simulink model "Plant"  (R2022b)
settings: Solver=FixedStepAuto  StartTime=start_time  StopTime=end_time  FixedStep=PLANT_CONST.dt  RelTol=1e-3  EnableMultiTasking=on
values from neighbouring files (symbols this model uses):
  PLANT_EXPORT = Simulink.Parameter(PLANT_EXPORT_VALUE)    [plant_model_init.m]
undefined symbols (not defined in the file or in its folder): acc_x, acc_x_O, acc_y, acc_y_O, acc_z, acc_z_O, alt, alt_0, DiscIntNeverNeededParam, fixType, gyr_x, gyr_y, gyr_z, h_R, hAcc, height, lat, lon, M_BO, M_OB, mag_x, mag_y, mag_z, numSV, phi, PLANT_CONST, psi, quat, rot_x_B, rot_y_B, rot_z_B, sAcc, Sensor_Model, temprature, theta, timestamp, vAcc, vel_x_O, vel_y_O, vel_z_O, velD, velE, velN, x_R, y_R
libraries: FMT_Model_Lib x9, dspsrcs4 x5, simulink_extras x1, autolibshared x1, simulink x1
(part 1 of 2)
settings Model: Creator=19114  LastModifiedBy=19114
settings OptimizationCC: DefaultParameterBehavior=Inlined  EnhancedBackFolding=on  PassReuseOutputArgsAs=Individual arguments  ZeroExternalMemoryAtStartup=off  ZeroInternalMemoryAtStartup=off  OptimizeBlockOrder=speed  DifferentSizesBufferReuse=on  OptimizationCustomize=off  EfficientTunableParamExpr=on
settings DebuggingCC: ParameterTunabilityLossMsg=error
settings SFSimCC: MATLABDynamicMemAlloc=off
settings RTWCC: Description=Embedded Coder  SystemTargetFile=ert.tlc  TemplateMakefile=ert_default_tmf
settings CodeAppCC: ForceParamTrailComments=on  IgnoreCustomStorageClasses=off  OperatorAnnotations=on  SimulinkDataObjDesc=on  SFDataObjDesc=on  InsertBlockDesc=on
settings ERTTargetCC: TargetLangStandard=C99 (ISO)  GenerateSampleERTMain=on  InlinedParameterPlacement=NonHierarchical  ERTCustomFileTemplate=example_file_process.tlc

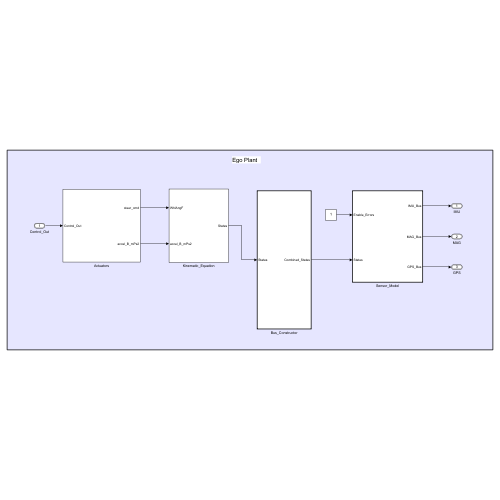
[thumbnail: Simulink's stored preview of the top-level diagram]
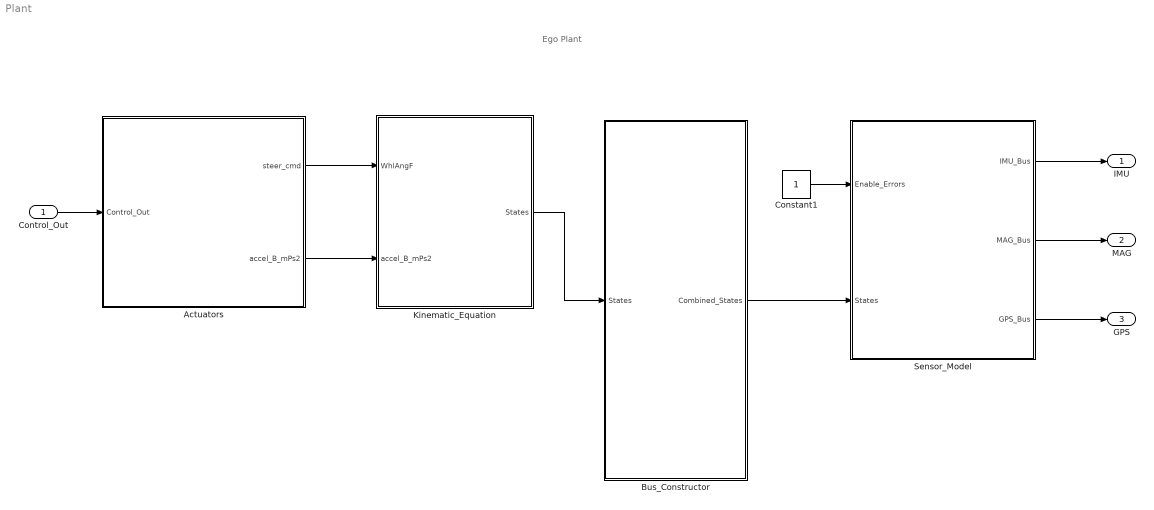
== system Plant ==
  note: Ego Plant
  Control_Out : Inport  OutDataTypeStr=Bus: Control_Out_Bus
  Actuators : Subsystem
  Bus_Constructor : Subsystem  TreatAsAtomicUnit=on  mask{lat_0=0.65673, lon_0=-2.1361, hgt_0=0}
      mask prompts: lat_0 "init latitude (rad)"; lon_0 "init lontitude (rad)"; hgt_0 "init height (m)"
  Constant1 : Constant  OutDataTypeStr=Inherit: Inherit via back propagation
  Kinematic_Equation : Subsystem
  Sensor_Model : Subsystem  TreatAsAtomicUnit=on
  IMU : Outport  OutDataTypeStr=Bus: IMU_Bus  VectorParamsAs1DForOutWhenUnconnected=off
  MAG : Outport  Port=2  OutDataTypeStr=Bus: MAG_Bus  VectorParamsAs1DForOutWhenUnconnected=off
  GPS : Outport  Port=3  OutDataTypeStr=Bus: GPS_uBlox_Bus  VectorParamsAs1DForOutWhenUnconnected=off
  wires:
  Control_Out/1 -> Actuators/1(Control_Out)
  Actuators/1(steer_cmd) -> Kinematic_Equation/1(WhlAngF)
  Kinematic_Equation/1(States) -> Bus_Constructor/1(States)
  Actuators/2(accel_B_mPs2) -> Kinematic_Equation/2(accel_B_mPs2)
  Constant1/1 -> Sensor_Model/1(Enable_Errors)
  Bus_Constructor/1(Combined_States) -> Sensor_Model/2(States)
  Sensor_Model/3(GPS_Bus) -> GPS/1
  Sensor_Model/2(MAG_Bus) -> MAG/1
  Sensor_Model/1(IMU_Bus) -> IMU/1

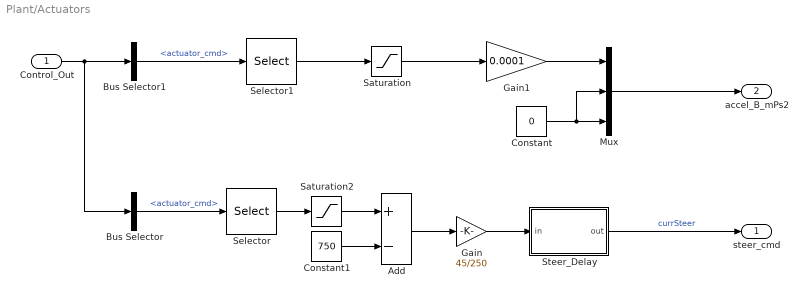
== system Plant/Actuators ==
  Control_Out : Inport
  Add : Sum  Inputs=+-  OutDataTypeStr=single
  Bus Selector : BusSelector  OutputSignals=actuator_cmd
  Bus Selector1 : BusSelector  OutputSignals=actuator_cmd
  Constant : Constant  Value=0  OutDataTypeStr=Inherit: Inherit via back propagation
  Constant1 : Constant  Value=750  OutDataTypeStr=int16
  Gain : Gain  Gain=45/250
  Gain1 : Gain  Gain=0.0001  OutDataTypeStr=single
  Mux : Mux  Inputs=3
  Saturation : Saturate  UpperLimit=10000  LowerLimit=-10000
  Saturation2 : Saturate  UpperLimit=1250  LowerLimit=250  OutDataTypeStr=int16
  Selector : Selector  InputPortWidth=4  IndexOptions=Index vector (dialog)  Indices=[1]  OutputSizes=1
  Selector1 : Selector  InputPortWidth=4  IndexOptions=Index vector (dialog)  Indices=[2]  OutputSizes=1
  Steer_Delay : Subsystem  mask{K=1, T=0.1}
      mask Display: disp('K/(1+Tz^{-1})', 'texmode', 'on')
  steer_cmd : Outport
  accel_B_mPs2 : Outport  Port=2  VectorParamsAs1DForOutWhenUnconnected=off
  wires:
  Bus Selector/1 -> Selector/1  "<actuator_cmd>"
  Control_Out/1 -> Bus Selector1/1, Bus Selector/1
  Selector/1 -> Saturation2/1
  Saturation2/1 -> Add/1
  Constant1/1 -> Add/2
  Add/1 -> Gain/1
  Gain/1 -> Steer_Delay/1(in)
  Steer_Delay/1(out) -> steer_cmd/1  "currSteer"
  Selector1/1 -> Saturation/1
  Saturation/1 -> Gain1/1
  Bus Selector1/1 -> Selector1/1  "<actuator_cmd>"
  Gain1/1 -> Mux/1
  Mux/1 -> accel_B_mPs2/1
  Constant/1 -> Mux/3, Mux/2

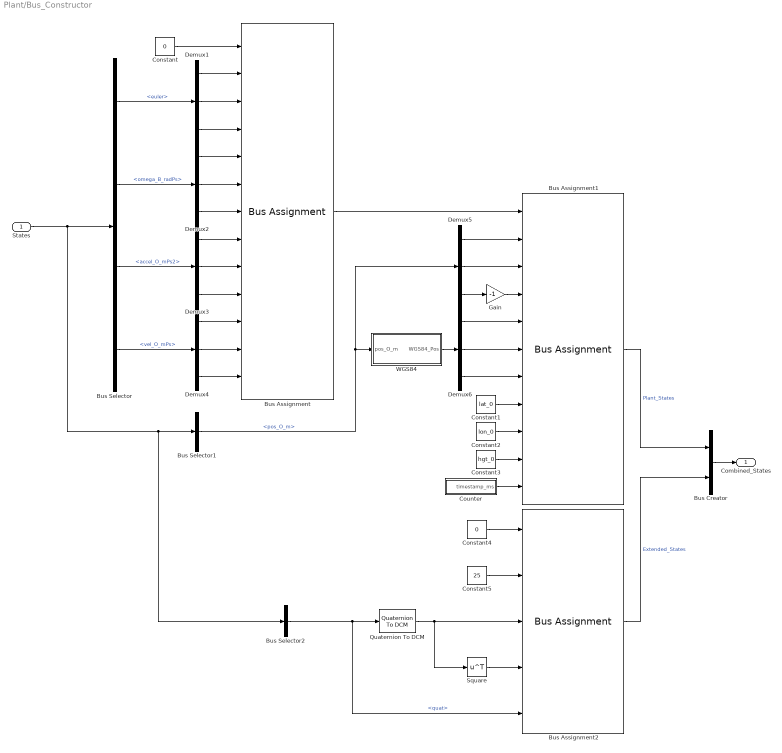
== system Plant/Bus_Constructor ==
  States : Inport
  Bus Assignment : BusAssignment  AssignedSignals=phi,theta,psi,rot_x_B,rot_y_B,rot_z_B,acc_x_O,acc_y_O,acc_z_O,vel_x_O,vel_y_O,vel_z_O
  Bus Assignment1 : BusAssignment  AssignedSignals=x_R,y_R,h_R,lat,lon,alt,lat_0,lon_0,alt_0,timestamp
  Bus Assignment2 : BusAssignment  AssignedSignals=temprature,M_BO,M_OB,quat
  Bus Creator : BusCreator  Inputs=2
  Bus Selector : BusSelector  OutputSignals=euler,omega_B_radPs,accel_O_mPs2,vel_O_mPs
  Bus Selector1 : BusSelector  OutputSignals=pos_O_m
  Bus Selector2 : BusSelector  OutputSignals=quat
  Constant : Constant  Value=0  OutDataTypeStr=Bus: Plant_States_Bus
  Constant1 : Constant  Value=lat_0
  Constant2 : Constant  Value=lon_0
  Constant3 : Constant  Value=hgt_0
  Constant4 : Constant  Value=0  OutDataTypeStr=Bus: Extended_States_Bus
  Constant5 : Constant  Value=25  OutDataTypeStr=Inherit: Inherit via back propagation
  Counter : Subsystem
  Demux{1..6} (6 alike) : Demux  Outputs=3
  Gain : Gain  Gain=-1  OutDataTypeStr=Inherit: Same as input
  Quaternion To DCM : FMT_Model_Lib/Quaternion/Quaternion To DCM
      settings: SourceProductName=FMT Toolbox
  Square : Math  Operator=transpose  SignedPower=on
  WGS84 : Subsystem
  Combined_States : Outport  VectorParamsAs1DForOutWhenUnconnected=off
  wires:
  Constant/1 -> Bus Assignment/1
  States/1 -> Bus Selector2/1, Bus Selector1/1, Bus Selector/1
  Bus Selector/1 -> Demux1/1  "<euler>"
  Bus Selector/2 -> Demux2/1  "<omega_B_radPs>"
  Bus Selector/3 -> Demux3/1  "<accel_O_mPs2>"
  Bus Selector/4 -> Demux4/1  "<vel_O_mPs>"
  Bus Assignment/1 -> Bus Assignment1/1
  Bus Selector1/1 -> Demux5/1, WGS84/1(pos_O_m)  "<pos_O_m>"
  Bus Assignment1/1 -> Bus Creator/1  "Plant_States"
  Demux1/2 -> Bus Assignment/3
  Demux5/3 -> Gain/1
  WGS84/1(WGS84_Pos) -> Demux6/1
  Demux1/1 -> Bus Assignment/2
  Demux1/3 -> Bus Assignment/4
  Demux2/1 -> Bus Assignment/5
  Demux2/2 -> Bus Assignment/6
  Demux2/3 -> Bus Assignment/7
  Demux3/1 -> Bus Assignment/8
  Demux3/2 -> Bus Assignment/9
  Demux3/3 -> Bus Assignment/10
  Demux4/1 -> Bus Assignment/11
  Demux4/2 -> Bus Assignment/12
  Demux4/3 -> Bus Assignment/13
  Demux5/2 -> Bus Assignment1/3
  Gain/1 -> Bus Assignment1/4
  Demux5/1 -> Bus Assignment1/2
  Demux6/1 -> Bus Assignment1/5
  Demux6/2 -> Bus Assignment1/6
  Demux6/3 -> Bus Assignment1/7
  Constant2/1 -> Bus Assignment1/9
  Constant1/1 -> Bus Assignment1/8
  Constant3/1 -> Bus Assignment1/10
  Constant4/1 -> Bus Assignment2/1
  Constant5/1 -> Bus Assignment2/2
  Bus Selector2/1 -> Bus Assignment2/5, Quaternion To DCM/1  "<quat>"
  Bus Assignment2/1 -> Bus Creator/2  "Extended_States"
  Bus Creator/1 -> Combined_States/1
  Counter/1(timestamp_ms) -> Bus Assignment1/11
  Square/1 -> Bus Assignment2/4
  Quaternion To DCM/1 -> Square/1, Bus Assignment2/3

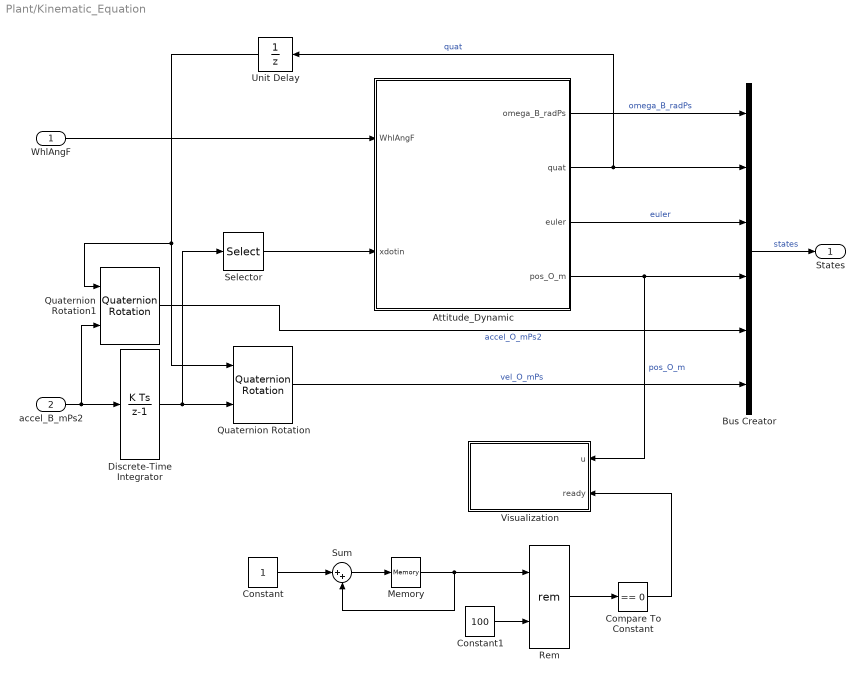
== system Plant/Kinematic_Equation ==
  WhlAngF : Inport
  accel_B_mPs2 : Inport  Port=2
  Attitude_Dynamic : Subsystem
  Bus Creator : BusCreator  Inputs=6
  Compare To Constant : simulink/Logic and Bit Operations/Compare To Constant  relop===  const=0  OutDataTypeStr=boolean
  Constant : Constant
  Constant1 : Constant  Value=100
  Discrete-Time Integrator : DiscreteIntegrator  InitialCondition=[0;0;0]  SampleTime=-1  ICPrevOutput=DiscIntNeverNeededParam  ICPrevScaledInput=DiscIntNeverNeededParam
  Memory : Memory
  Quaternion Rotation : FMT_Model_Lib/Quaternion/Quaternion Rotation
      settings: SourceProductName=FMT Toolbox
  Quaternion Rotation1 : FMT_Model_Lib/Quaternion/Quaternion Rotation
      settings: SourceProductName=FMT Toolbox
  Rem : Math  Operator=rem
  Selector : Selector  InputPortWidth=3  IndexOptions=Index vector (dialog)  Indices=[1]  OutputSizes=1
  Sum : Sum  Inputs=|++
  Unit Delay : UnitDelay  InitialCondition=[1 0 0 0]  SampleTime=-1  HasFrameUpgradeWarning=on
  Visualization : MATLAB Function  TreatAsAtomicUnit=on
  States : Outport  VectorParamsAs1DForOutWhenUnconnected=off
  wires:
  Attitude_Dynamic/1(omega_B_radPs) -> Bus Creator/1  "omega_B_radPs"
  Bus Creator/1 -> States/1  "states"
  WhlAngF/1 -> Attitude_Dynamic/1(WhlAngF)
  Attitude_Dynamic/2(quat) -> Unit Delay/1, Bus Creator/2  "quat"
  Attitude_Dynamic/3(euler) -> Bus Creator/3  "euler"
  Unit Delay/1 -> Quaternion Rotation1/1, Quaternion Rotation/1
  Selector/1 -> Attitude_Dynamic/2(xdotin)
  Quaternion Rotation/1 -> Bus Creator/6  "vel_O_mPs"
  accel_B_mPs2/1 -> Quaternion Rotation1/2, Discrete-Time Integrator/1
  Quaternion Rotation1/1 -> Bus Creator/5  "accel_O_mPs2"
  Attitude_Dynamic/4(pos_O_m) -> Visualization/1(u), Bus Creator/4  "pos_O_m"
  Memory/1 -> Rem/1, Sum/2
  Constant1/1 -> Rem/2
  Rem/1 -> Compare To Constant/1
  Compare To Constant/1 -> Visualization/2(ready)
  Constant/1 -> Sum/1
  Sum/1 -> Memory/1
  Discrete-Time Integrator/1 -> Quaternion Rotation/2, Selector/1

== system Plant/Sensor_Model ==
  Enable_Errors : Inport  OutDataTypeStr=uint8
  States : Inport  Port=2
  Counter : Subsystem
  Sensor_GPS : Subsystem  TreatAsAtomicUnit=on
  Sensor_IMU : Subsystem  TreatAsAtomicUnit=on
  Sensor_MAG : Subsystem  TreatAsAtomicUnit=on
  IMU_Bus : Outport  VectorParamsAs1DForOutWhenUnconnected=off
  MAG_Bus : Outport  Port=2  VectorParamsAs1DForOutWhenUnconnected=off
  GPS_Bus : Outport  Port=3  VectorParamsAs1DForOutWhenUnconnected=off
  wires:
  Counter/1(timestamp_ms) -> Sensor_MAG/3(timestamp_ms), Sensor_IMU/3(timestamp_ms), Sensor_GPS/3(timestamp_ms)
  States/1 -> Sensor_GPS/1(States), Sensor_MAG/1(States), Sensor_IMU/1(States)
  Sensor_MAG/1(MAG_Bus) -> MAG_Bus/1
  Sensor_IMU/1(IMU_Bus) -> IMU_Bus/1
  Enable_Errors/1 -> Sensor_IMU/2(Enable_Errors), Sensor_GPS/2(Enable_Errors), Sensor_MAG/2(Enable_Errors)
  Sensor_GPS/1(GPS_Bus) -> GPS_Bus/1

== system Plant/Actuators/Steer_Delay ==
  in : Inport
  Discrete-Time Integrator : DiscreteIntegrator  gainval=K  SampleTime=-1  ICPrevOutput=DiscIntNeverNeededParam  ICPrevScaledInput=DiscIntNeverNeededParam
  Gain : Gain  Gain=1/T
  Subtract : Sum  Inputs=+-  OutDataTypeStr=single
  out : Outport  VectorParamsAs1DForOutWhenUnconnected=off
  wires:
  in/1 -> Subtract/1
  Subtract/1 -> Gain/1
  Gain/1 -> Discrete-Time Integrator/1
  Discrete-Time Integrator/1 -> Subtract/2, out/1

== system Plant/Bus_Constructor/Counter ==
  Data Type Conversion2 : DataTypeConversion  OutDataTypeStr=uint32  SaturateOnIntegerOverflow=off  RndMeth=Floor
  Delay : Delay  DelayLength=1  InitialCondition=0
  Sum : Sum  Inputs=|++
  dt : Constant  Value=PLANT_EXPORT.period  OutDataTypeStr=uint32
  timestamp_ms : Outport  VectorParamsAs1DForOutWhenUnconnected=off
  wires:
  dt/1 -> Sum/1
  Sum/1 -> Delay/1
  Delay/1 -> Data Type Conversion2/1
  Data Type Conversion2/1 -> timestamp_ms/1, Sum/2

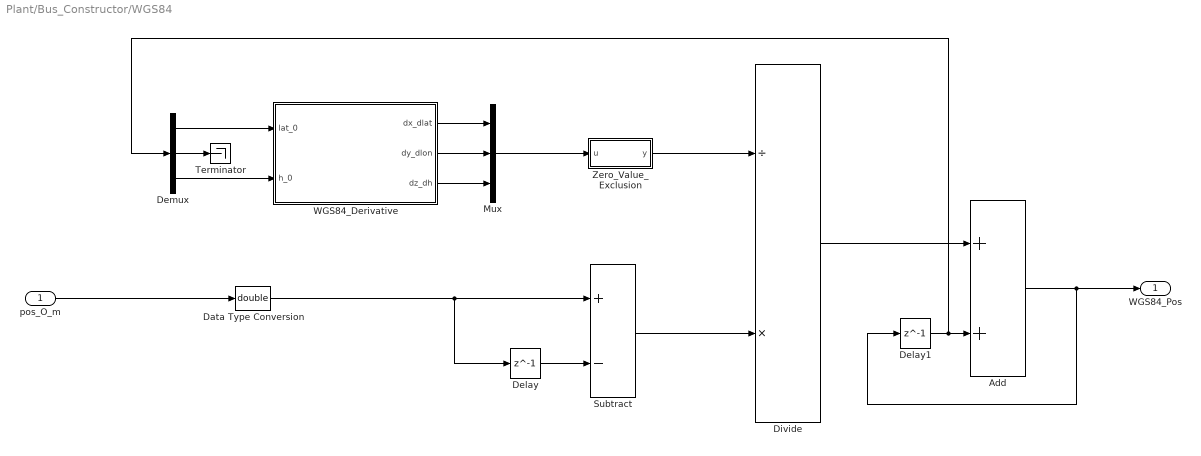
== system Plant/Bus_Constructor/WGS84 ==
  pos_O_m : Inport
  Add : Sum
  Data Type Conversion : DataTypeConversion  OutDataTypeStr=double  SaturateOnIntegerOverflow=off  RndMeth=Floor
  Delay : Delay  DelayLength=1
  Delay1 : Delay  DelayLength=1  InitialCondition=[lat_0;lon_0;hgt_0]
  Demux : Demux  Outputs=3
  Divide : Product  Inputs=/*
  Mux : Mux  Inputs=3
  Subtract : Sum  Inputs=+-
  Terminator : Terminator
  WGS84_Derivative : Subsystem
  Zero_Value_Exclusion : Subsystem
  WGS84_Pos : Outport  VectorParamsAs1DForOutWhenUnconnected=off
  wires:
  pos_O_m/1 -> Data Type Conversion/1
  Delay/1 -> Subtract/2
  WGS84_Derivative/1(dx_dlat) -> Mux/1
  Mux/1 -> Zero_Value_Exclusion/1(u)
  Zero_Value_Exclusion/1(y) -> Divide/1
  WGS84_Derivative/3(dz_dh) -> Mux/3
  WGS84_Derivative/2(dy_dlon) -> Mux/2
  Subtract/1 -> Divide/2
  Divide/1 -> Add/1
  Delay1/1 -> Demux/1, Add/2
  Add/1 -> Delay1/1, WGS84_Pos/1
  Demux/1 -> WGS84_Derivative/1(lat_0)
  Demux/3 -> WGS84_Derivative/2(h_0)
  Demux/2 -> Terminator/1
  Data Type Conversion/1 -> Delay/1, Subtract/1

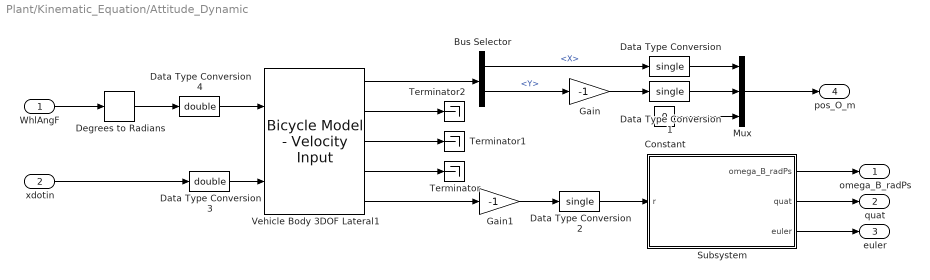
== system Plant/Kinematic_Equation/Attitude_Dynamic ==
  WhlAngF : Inport
  xdotin : Inport  Port=2
  Bus Selector : BusSelector  OutputSignals=InertFrm.RearAxl.Disp.X,InertFrm.RearAxl.Disp.Y
  Constant : Constant  Value=0  OutDataTypeStr=Inherit: Inherit via back propagation
  Data Type Conversion : DataTypeConversion  OutDataTypeStr=single  SaturateOnIntegerOverflow=off  RndMeth=Floor
  Data Type Conversion1 : DataTypeConversion  OutDataTypeStr=single  SaturateOnIntegerOverflow=off  RndMeth=Floor
  Data Type Conversion2 : DataTypeConversion  OutDataTypeStr=single  SaturateOnIntegerOverflow=off  RndMeth=Floor
  Data Type Conversion3 : DataTypeConversion  OutDataTypeStr=double  SaturateOnIntegerOverflow=off  RndMeth=Floor
  Data Type Conversion4 : DataTypeConversion  OutDataTypeStr=double  SaturateOnIntegerOverflow=off  RndMeth=Floor
  Degrees to Radians : simulink_extras/Transformations/Degrees to Radians
  Gain : Gain  Gain=-1
  Gain1 : Gain  Gain=-1
  Mux : Mux  Inputs=3
  Subsystem : Subsystem
  Terminator : Terminator
  Terminator1 : Terminator
  Terminator2 : Terminator
  Vehicle Body 3DOF Lateral1 : autolibshared/Bicycle Model - Velocity Input  trackMode=Single (bicycle)  inputMode=External longitudinal forces  frontSteerMode=on  rearSteerMode=off  windMode=off  muMode=off  extFMode=off  extMMode=off  aMode=3  NF=2  NR=2  m=1575  a=1.2  b=1.6  h=0.35  X_o=0  xdot_o=0  CalphaMode=off  sigmaMode=on  w=[1.4,1.4]  Cy_f=19e3  Cy_r=20e3  sigma_f=.1  sigma_r=.1  alpha_f_brk=[-.1 .1]  Cy_f_data=[-9e3 9e3]  alpha_r_brk=[-.1 .1]  Cy_r_data=[-9e3 9e3]  Y_o=0  ydot_o=0  Izz=4000  psi_o=0  r_o=0  Af=2  Cd=.3  Cl=.1  Cpm=.1  beta_w=[0:0.01:0.3]  Cs=[0:0.03:0.9]  Cym=[0:0.01:0.3]  Pabs=101325  Tair=273  g=9.81  mu=1  xdot_tol=0.01  Fznom=5000  Fxtire_sat=1e6  Fytire_sat=1e6  longOff=0  latOff=0  vertOff=0
  omega_B_radPs : Outport
  quat : Outport  Port=2
  euler : Outport  Port=3
  pos_O_m : Outport  Port=4
  wires:
  Vehicle Body 3DOF Lateral1/4 -> Terminator/1
  Vehicle Body 3DOF Lateral1/3 -> Terminator1/1
  Subsystem/1(omega_B_radPs) -> omega_B_radPs/1
  Subsystem/2(quat) -> quat/1
  Subsystem/3(euler) -> euler/1
  Bus Selector/2 -> Gain/1  "<Y>"
  Bus Selector/1 -> Data Type Conversion/1  "<X>"
  Vehicle Body 3DOF Lateral1/2 -> Terminator2/1
  Constant/1 -> Mux/3
  Mux/1 -> pos_O_m/1
  Vehicle Body 3DOF Lateral1/1 -> Bus Selector/1
  Data Type Conversion/1 -> Mux/1
  Gain/1 -> Data Type Conversion1/1
  Data Type Conversion1/1 -> Mux/2
  Data Type Conversion2/1 -> Subsystem/1(r)
  xdotin/1 -> Data Type Conversion3/1
  WhlAngF/1 -> Degrees to Radians/1
  Data Type Conversion3/1 -> Vehicle Body 3DOF Lateral1/2
  Data Type Conversion4/1 -> Vehicle Body 3DOF Lateral1/1
  Vehicle Body 3DOF Lateral1/5 -> Gain1/1
  Degrees to Radians/1 -> Data Type Conversion4/1
  Gain1/1 -> Data Type Conversion2/1

== system Plant/Sensor_Model/Counter ==
  Data Type Conversion2 : DataTypeConversion  OutDataTypeStr=uint32  SaturateOnIntegerOverflow=off  RndMeth=Floor
  Memory1 : Memory
  Sum : Sum  Inputs=|++
  dt : Constant  Value=PLANT_EXPORT.period  OutDataTypeStr=uint32
  timestamp_ms : Outport  VectorParamsAs1DForOutWhenUnconnected=off
  wires:
  dt/1 -> Sum/1
  Sum/1 -> Memory1/1
  Memory1/1 -> Sum/2, Data Type Conversion2/1
  Data Type Conversion2/1 -> timestamp_ms/1

== system Plant/Sensor_Model/Sensor_GPS ==
  States : Inport
  Enable_Errors : Inport  Port=2
  timestamp_ms : Inport  Port=3
  Bus_Constructor : Subsystem
  GPS : Subsystem
  GPS_Bus : Outport  VectorParamsAs1DForOutWhenUnconnected=off
  wires:
  Bus_Constructor/1(GPS_Bus) -> GPS_Bus/1
  timestamp_ms/1 -> Bus_Constructor/2(timestamp_ms)
  Enable_Errors/1 -> GPS/1(Enable_Errors)
  States/1 -> GPS/2(States)
  GPS/1(GPS_Raw) -> Bus_Constructor/1(GPS_Raw)

== system Plant/Sensor_Model/Sensor_IMU ==
  States : Inport
  Enable_Errors : Inport  Port=2
  timestamp_ms : Inport  Port=3
  Accelerometer : Subsystem
  Bus_Constructor : Subsystem
  Gyroscope : Subsystem
  IMU_Bus : Outport  VectorParamsAs1DForOutWhenUnconnected=off
  wires:
  Gyroscope/1(Gyro_Raw) -> Bus_Constructor/1(Gyro_Raw)
  Bus_Constructor/1(IMU_Bus) -> IMU_Bus/1
  States/1 -> Gyroscope/1(States), Accelerometer/1(States)
  Enable_Errors/1 -> Gyroscope/2(Enable_Errors), Accelerometer/2(Enable_Errors)
  Accelerometer/1(Acc_Raw) -> Bus_Constructor/2(Acc_Raw)
  timestamp_ms/1 -> Bus_Constructor/3(timestamp_ms)

== system Plant/Sensor_Model/Sensor_MAG ==
  States : Inport
  Enable_Errors : Inport  Port=2
  timestamp_ms : Inport  Port=3
  Bus_Constructor : Subsystem
  Magnetometer : Subsystem
  MAG_Bus : Outport  VectorParamsAs1DForOutWhenUnconnected=off
  wires:
  Magnetometer/1(Mag_Raw) -> Bus_Constructor/1(Mag_Raw)
  Bus_Constructor/1(MAG_Bus) -> MAG_Bus/1
  States/1 -> Magnetometer/1(States)
  Enable_Errors/1 -> Magnetometer/2(Enable_Errors)
  timestamp_ms/1 -> Bus_Constructor/2(timestamp_ms)

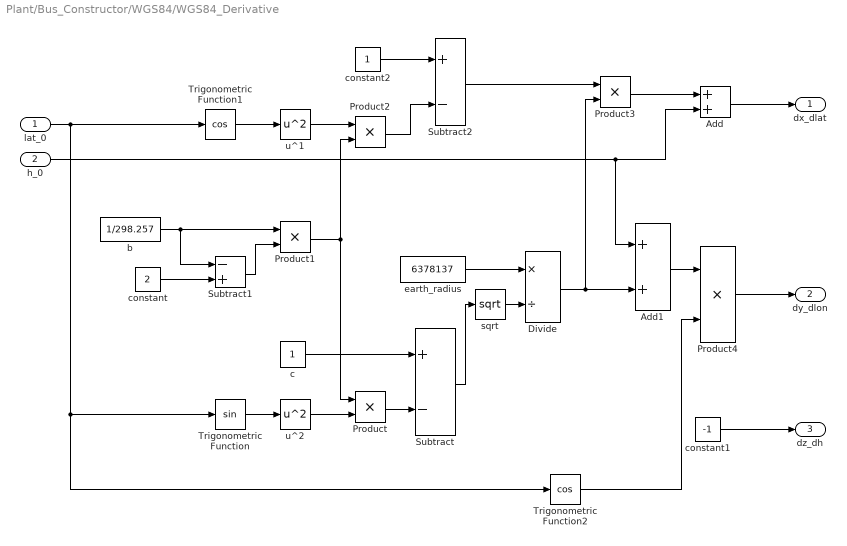
== system Plant/Bus_Constructor/WGS84/WGS84_Derivative ==
  lat_0 : Inport
  h_0 : Inport  Port=2
  Add : Sum
  Add1 : Sum
  Divide : Product  Inputs=*/
  Product{,1..4} (5 alike) : Product  RndMeth=Zero
  Subtract : Sum  Inputs=+-
  Subtract1 : Sum  Inputs=-+
  Subtract2 : Sum  Inputs=+-
  Trigonometric Function : Trigonometry
  Trigonometric Function1 : Trigonometry  Operator=cos
  Trigonometric Function2 : Trigonometry  Operator=cos
  b : Constant  Value=1/298.257
  c : Constant
  constant : Constant  Value=2
  constant1 : Constant  Value=-1
  constant2 : Constant
  earth_radius : Constant  Value=6378137
  sqrt : Math  Operator=sqrt  SignedPower=on
  u^1 : Math  Operator=square  SignedPower=on
  u^2 : Math  Operator=square  SignedPower=on
  dx_dlat : Outport  VectorParamsAs1DForOutWhenUnconnected=off
  dy_dlon : Outport  Port=2  VectorParamsAs1DForOutWhenUnconnected=off
  dz_dh : Outport  Port=3  InitialOutput=1  VectorParamsAs1DForOutWhenUnconnected=off
  wires:
  constant1/1 -> dz_dh/1
  Product4/1 -> dy_dlon/1
  Add1/1 -> Product4/1
  Trigonometric Function2/1 -> Product4/2
  Product3/1 -> Add/1
  Subtract2/1 -> Product3/1
  Product2/1 -> Subtract2/2
  u^1/1 -> Product2/1
  Trigonometric Function1/1 -> u^1/1
  constant2/1 -> Subtract2/1
  h_0/1 -> Add1/1, Add/2
  Add/1 -> dx_dlat/1
  Divide/1 -> Product3/2, Add1/2
  sqrt/1 -> Divide/2
  Product1/1 -> Product2/2, Product/1
  Subtract1/1 -> Product1/2
  constant/1 -> Subtract1/2
  b/1 -> Subtract1/1, Product1/1
  Product/1 -> Subtract/2
  Subtract/1 -> sqrt/1
  c/1 -> Subtract/1
  u^2/1 -> Product/2
  Trigonometric Function/1 -> u^2/1
  lat_0/1 -> Trigonometric Function2/1, Trigonometric Function/1, Trigonometric Function1/1
  earth_radius/1 -> Divide/1

== system Plant/Bus_Constructor/WGS84/Zero_Value_Exclusion ==
  u : Inport
  Abs : Abs  SaturateOnIntegerOverflow=off
  Constant : Constant
  Product : Product  RndMeth=Zero
  Saturation : Saturate  UpperLimit=10e7  LowerLimit=1e-6  LinearizeAsGain=off
  Sign : Signum
  Switch : Switch  Criteria=u2 ~= 0  SaturateOnIntegerOverflow=off  InputSameDT=off
  y : Outport  VectorParamsAs1DForOutWhenUnconnected=off
  wires:
  u/1 -> Sign/1, Abs/1
  Abs/1 -> Saturation/1
  Saturation/1 -> Product/1
  Sign/1 -> Switch/2, Switch/1
  Product/1 -> y/1
  Switch/1 -> Product/2
  Constant/1 -> Switch/3

== system Plant/Kinematic_Equation/Attitude_Dynamic/Subsystem ==
  r : Inport
  Constant : Constant  Value=0  OutDataTypeStr=Inherit: Inherit via back propagation
  Constant2 : Constant  Value=0  OutDataTypeStr=Inherit: Inherit via back propagation
  Mux : Mux  Inputs=3
  Quaternion To Euler : FMT_Model_Lib/Quaternion/Quaternion To Euler
      settings: SourceProductName=FMT Toolbox
  Quaternuin_Update : Subsystem
  quat0 : Constant  Value=[1;0;0;0]  OutDataTypeStr=single
  omega_B_radPs : Outport
  quat : Outport  Port=2
  euler : Outport  Port=3
  wires:
  Quaternuin_Update/1(quat) -> quat/1, Quaternion To Euler/1
  Constant2/1 -> Mux/1, Mux/2
  Quaternion To Euler/1 -> euler/1
  r/1 -> Mux/3
  Mux/1 -> omega_B_radPs/1, Quaternuin_Update/1(omega_B_radPs)
  Constant/1 -> Quaternuin_Update/2(reset)
  quat0/1 -> Quaternuin_Update/3(init_quat)

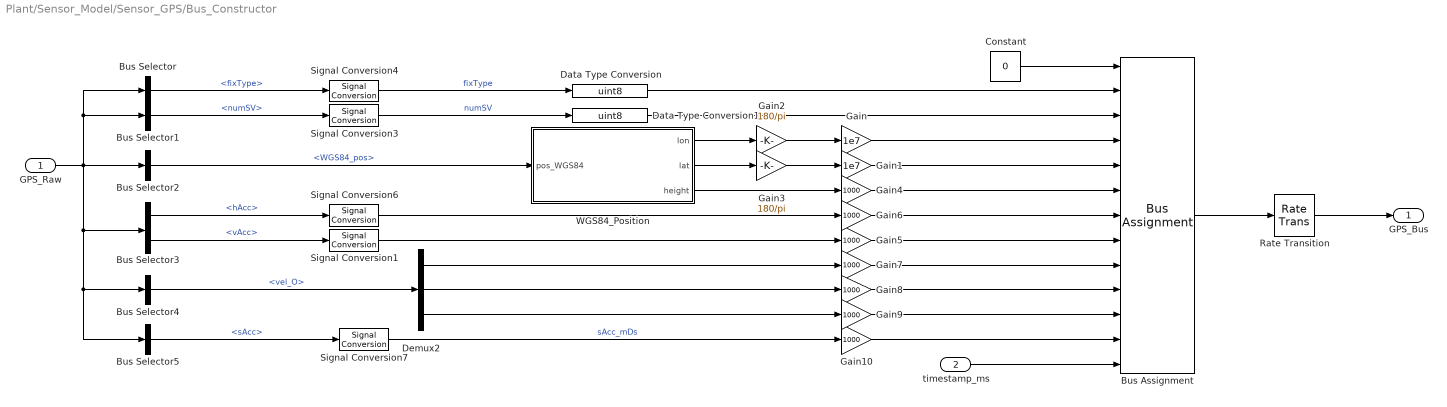
== system Plant/Sensor_Model/Sensor_GPS/Bus_Constructor ==
  GPS_Raw : Inport
  timestamp_ms : Inport  Port=2
  Bus Assignment : BusAssignment  AssignedSignals=fixType,numSV,lon,lat,height,hAcc,vAcc,velN,velE,velD,sAcc,timestamp
  Bus Selector : BusSelector  OutputSignals=fixType
  Bus Selector1 : BusSelector  OutputSignals=numSV
  Bus Selector2 : BusSelector  OutputSignals=WGS84_pos
  Bus Selector3 : BusSelector  OutputSignals=hAcc,vAcc
  Bus Selector4 : BusSelector  OutputSignals=vel_O
  Bus Selector5 : BusSelector  OutputSignals=sAcc
  Constant : Constant  Value=0  OutDataTypeStr=Bus: GPS_uBlox_Bus
  Data Type Conversion : DataTypeConversion  OutDataTypeStr=uint8  SaturateOnIntegerOverflow=off  RndMeth=Floor
  Data Type Conversion1 : DataTypeConversion  OutDataTypeStr=uint8  SaturateOnIntegerOverflow=off  RndMeth=Floor
  Demux2 : Demux  Outputs=3
  Gain : Gain  Gain=1e7  OutDataTypeStr=int32
      settings: AttributesFormatString=Gain: %<Gain>
  Gain1 : Gain  Gain=1e7  OutDataTypeStr=int32
      settings: AttributesFormatString=Gain: %<Gain>
  Gain10 : Gain  Gain=1000  OutDataTypeStr=uint32
      settings: AttributesFormatString=Gain: %<Gain>
  Gain2 : Gain  Gain=180/pi
      settings: AttributesFormatString=Gain: %<Gain>
  Gain3 : Gain  Gain=180/pi
      settings: AttributesFormatString=Gain: %<Gain>
  Gain{4,7..9} (4 alike) : Gain  Gain=1000  OutDataTypeStr=int32
      settings: AttributesFormatString=Gain: %<Gain>
  Gain5 : Gain  Gain=1000  OutDataTypeStr=uint32
      settings: AttributesFormatString=Gain: %<Gain>
  Gain6 : Gain  Gain=1000  OutDataTypeStr=uint32
      settings: AttributesFormatString=Gain: %<Gain>
  Rate Transition : RateTransition  OutPortSampleTime=0.1
  Signal Conversion{1,3..4,6..7} (5 alike) : SignalConversion  OverrideOpt=off
  WGS84_Position : Subsystem
  GPS_Bus : Outport  VectorParamsAs1DForOutWhenUnconnected=off
  wires:
  Bus Selector5/1 -> Signal Conversion7/1  "<sAcc>"
  Bus Selector3/1 -> Signal Conversion6/1  "<hAcc>"
  Bus Selector1/1 -> Signal Conversion3/1  "<numSV>"
  Bus Selector4/1 -> Demux2/1  "<vel_O>"
  Gain5/1 -> Bus Assignment/8
  Data Type Conversion/1 -> Bus Assignment/2
  Gain4/1 -> Bus Assignment/6
  Gain3/1 -> Gain1/1
  Signal Conversion6/1 -> Gain6/1
  Gain6/1 -> Bus Assignment/7
  Gain8/1 -> Bus Assignment/10
  Gain7/1 -> Bus Assignment/9
  Gain10/1 -> Bus Assignment/12
  Constant/1 -> Bus Assignment/1
  Gain2/1 -> Gain/1
  Bus Assignment/1 -> Rate Transition/1
  Gain9/1 -> Bus Assignment/11
  Gain/1 -> Bus Assignment/4
  Data Type Conversion1/1 -> Bus Assignment/3
  Gain1/1 -> Bus Assignment/5
  Signal Conversion7/1 -> Gain10/1  "sAcc_mDs"
  Demux2/1 -> Gain7/1
  Demux2/2 -> Gain8/1
  Demux2/3 -> Gain9/1
  Bus Selector2/1 -> WGS84_Position/1(pos_WGS84)  "<WGS84_pos>"
  WGS84_Position/1(lon) -> Gain2/1
  WGS84_Position/2(lat) -> Gain3/1
  WGS84_Position/3(height) -> Gain4/1
  Signal Conversion3/1 -> Data Type Conversion1/1  "numSV"
  Signal Conversion4/1 -> Data Type Conversion/1  "fixType"
  Bus Selector3/2 -> Signal Conversion1/1  "<vAcc>"
  Signal Conversion1/1 -> Gain5/1
  Rate Transition/1 -> GPS_Bus/1
  timestamp_ms/1 -> Bus Assignment/13
  GPS_Raw/1 -> Bus Selector5/1, Bus Selector4/1, Bus Selector3/1, Bus Selector2/1, Bus Selector1/1, Bus Selector/1
  Bus Selector/1 -> Signal Conversion4/1  "<fixType>"

== system Plant/Sensor_Model/Sensor_GPS/GPS ==
  Enable_Errors : Inport
  States : Inport  Port=2
  Bus_Constructor : Subsystem
  Physical_Model : Subsystem
  Sensor_Model : Subsystem
  GPS_Raw : Outport  VectorParamsAs1DForOutWhenUnconnected=off
  wires:
  Physical_Model/1(WGS84_pos_rad) -> Sensor_Model/2(WGS84_pos_rad)
  Physical_Model/2(vel_O_mPs) -> Sensor_Model/3(vel_O_mPs)
  States/1 -> Physical_Model/1(States)
  Enable_Errors/1 -> Sensor_Model/1(Enable_Errors)
  Sensor_Model/1(WGS84_pos_meas) -> Bus_Constructor/1(WGS84_pos_meas)
  Sensor_Model/2(vel_O_meas) -> Bus_Constructor/2(vel_O_meas)
  Sensor_Model/3(numSV) -> Bus_Constructor/3(numSV)
  Sensor_Model/4(fixType) -> Bus_Constructor/4(fixType)
  Sensor_Model/5(h_Acc_m) -> Bus_Constructor/5(h_Acc_m)
  Sensor_Model/6(v_Acc_m) -> Bus_Constructor/6(v_Acc_m)
  Sensor_Model/7(s_Acc_mDs) -> Bus_Constructor/7(s_Acc_mDs)
  Bus_Constructor/1(GPS_Raw) -> GPS_Raw/1

== system Plant/Sensor_Model/Sensor_IMU/Accelerometer ==
  States : Inport
  Enable_Errors : Inport  Port=2
  Bus_Constructor : Subsystem
  Physical_Model : Subsystem
  Sensor_Model : Subsystem
  Acc_Raw : Outport  VectorParamsAs1DForOutWhenUnconnected=off
  wires:
  Sensor_Model/1(y) -> Bus_Constructor/1(Output)
  States/1 -> Physical_Model/1(States)
  Physical_Model/1(sfor_B_mPs2) -> Sensor_Model/2(u)
  Bus_Constructor/1(Acc_Raw) -> Acc_Raw/1
  Enable_Errors/1 -> Sensor_Model/1(Enable_Errors)

== system Plant/Sensor_Model/Sensor_IMU/Bus_Constructor ==
  Gyro_Raw : Inport
  Acc_Raw : Inport  Port=2
  timestamp_ms : Inport  Port=3
  Bus Assignment : BusAssignment  AssignedSignals=timestamp,gyr_x,gyr_y,gyr_z,acc_x,acc_y,acc_z
  Bus Selector : BusSelector  OutputSignals=Gyro_x_radPs,Gyro_y_radPs,Gyro_z_radPs
  Bus Selector1 : BusSelector  OutputSignals=Acc_x_mPs2,Acc_y_mPs2,Acc_z_mPs2
  Constant : Constant  Value=0  OutDataTypeStr=Bus: IMU_Bus
  IMU_Bus : Outport  VectorParamsAs1DForOutWhenUnconnected=off
  wires:
  Gyro_Raw/1 -> Bus Selector/1
  Acc_Raw/1 -> Bus Selector1/1
  Constant/1 -> Bus Assignment/1
  timestamp_ms/1 -> Bus Assignment/2
  Bus Assignment/1 -> IMU_Bus/1
  Bus Selector/1 -> Bus Assignment/3  "<Gyro_x_radPs>"
  Bus Selector/2 -> Bus Assignment/4  "<Gyro_y_radPs>"
  Bus Selector/3 -> Bus Assignment/5  "<Gyro_z_radPs>"
  Bus Selector1/1 -> Bus Assignment/6  "<Acc_x_mPs2>"
  Bus Selector1/2 -> Bus Assignment/7  "<Acc_y_mPs2>"
  Bus Selector1/3 -> Bus Assignment/8  "<Acc_z_mPs2>"

== system Plant/Sensor_Model/Sensor_IMU/Gyroscope ==
  States : Inport
  Enable_Errors : Inport  Port=2
  Bus_Constructor : Subsystem
  Physical_Model : Subsystem
  Sensor_Model : Subsystem
  Gyro_Raw : Outport  VectorParamsAs1DForOutWhenUnconnected=off
  wires:
  States/1 -> Physical_Model/1(States)
  Sensor_Model/1(y) -> Bus_Constructor/1(Output)
  Bus_Constructor/1(Gyro_Raw) -> Gyro_Raw/1
  Enable_Errors/1 -> Sensor_Model/1(Enable_Errors)
  Physical_Model/1(gyr_B_radDs) -> Sensor_Model/2(u)

== system Plant/Sensor_Model/Sensor_MAG/Bus_Constructor ==
  Mag_Raw : Inport
  timestamp_ms : Inport  Port=2
  Bus Assignment : BusAssignment  AssignedSignals=timestamp,mag_x,mag_y,mag_z
  Bus Selector : BusSelector  OutputSignals=Mag_x_gauss,Mag_y_gauss,Mag_z_gauss
  Constant : Constant  Value=0  OutDataTypeStr=Bus: MAG_Bus
  Rate Transition : RateTransition  OutPortSampleTime=0.01
  MAG_Bus : Outport  VectorParamsAs1DForOutWhenUnconnected=off
  wires:
  Bus Assignment/1 -> Rate Transition/1
  Constant/1 -> Bus Assignment/1
  timestamp_ms/1 -> Bus Assignment/2
  Rate Transition/1 -> MAG_Bus/1
  Bus Selector/1 -> Bus Assignment/3  "<Mag_x_gauss>"
  Mag_Raw/1 -> Bus Selector/1
  Bus Selector/2 -> Bus Assignment/4  "<Mag_y_gauss>"
  Bus Selector/3 -> Bus Assignment/5  "<Mag_z_gauss>"

== system Plant/Sensor_Model/Sensor_MAG/Magnetometer ==
  States : Inport
  Enable_Errors : Inport  Port=2
  Bus_Constructor : Subsystem
  Physical_Model : Subsystem
  Sensor_Model : Subsystem
  Mag_Raw : Outport  VectorParamsAs1DForOutWhenUnconnected=off
  wires:
  Bus_Constructor/1(Mag_Raw) -> Mag_Raw/1
  Sensor_Model/1(y) -> Bus_Constructor/1(Output)
  States/1 -> Physical_Model/1(States)
  Physical_Model/1(mag_B_gauss) -> Sensor_Model/2(u)
  Enable_Errors/1 -> Sensor_Model/1(Enable_Errors)

== system Plant/Kinematic_Equation/Attitude_Dynamic/Subsystem/Quaternuin_Update ==
  omega_B_radPs : Inport
  reset : Inport  Port=2
  init_quat : Inport  Port=3
  Discrete-Time Integrator : DiscreteIntegrator  ExternalReset=level  InitialConditionSource=external  SampleTime=-1  ICPrevOutput=DiscIntNeverNeededParam  ICPrevScaledInput=DiscIntNeverNeededParam
  Gain : Gain  Gain=0.5  OutDataTypeStr=Inherit: Same as input
  Multiply : Product  Multiplication=Matrix(*)  OutDataTypeStr=Inherit: Same as first input
  Quaternion_Update_Maxtrix : Subsystem
  quat : Outport  VectorParamsAs1DForOutWhenUnconnected=off
  wires:
  Gain/1 -> Discrete-Time Integrator/1  "dot_q"
  Discrete-Time Integrator/1 -> quat/1, Multiply/2
  init_quat/1 -> Discrete-Time Integrator/3
  reset/1 -> Discrete-Time Integrator/2
  Multiply/1 -> Gain/1
  Quaternion_Update_Maxtrix/1(W) -> Multiply/1
  omega_B_radPs/1 -> Quaternion_Update_Maxtrix/1(omega_B_radPs)

== system Plant/Sensor_Model/Sensor_GPS/Bus_Constructor/WGS84_Position ==
  pos_WGS84 : Inport
  Demux1 : Demux  Outputs=3
  Signal Conversion : SignalConversion  OverrideOpt=off
  Signal Conversion1 : SignalConversion  OverrideOpt=off
  Signal Conversion2 : SignalConversion  OverrideOpt=off
  lon : Outport  VectorParamsAs1DForOutWhenUnconnected=off
  lat : Outport  Port=2  VectorParamsAs1DForOutWhenUnconnected=off
  height : Outport  Port=3  VectorParamsAs1DForOutWhenUnconnected=off
  wires:
  Demux1/3 -> Signal Conversion2/1  "POS_h_WGS84"
  Signal Conversion/1 -> lon/1
  Demux1/1 -> Signal Conversion/1  "POS_lon_WGS84"
  pos_WGS84/1 -> Demux1/1
  Demux1/2 -> Signal Conversion1/1  "POS_lat_WGS84"
  Signal Conversion1/1 -> lat/1
  Signal Conversion2/1 -> height/1

== system Plant/Sensor_Model/Sensor_GPS/GPS/Bus_Constructor ==
  WGS84_pos_meas : Inport
  vel_O_meas : Inport  Port=2
  numSV : Inport  Port=3
  fixType : Inport  Port=4
  h_Acc_m : Inport  Port=5
  v_Acc_m : Inport  Port=6
  s_Acc_mDs : Inport  Port=7
  Bus Creator : BusCreator  Inputs=7
  GPS_Raw : Outport  VectorParamsAs1DForOutWhenUnconnected=off
  wires:
  WGS84_pos_meas/1 -> Bus Creator/1  "WGS84_pos"
  vel_O_meas/1 -> Bus Creator/2  "vel_O"
  numSV/1 -> Bus Creator/3  "numSV"
  fixType/1 -> Bus Creator/4  "fixType"
  h_Acc_m/1 -> Bus Creator/5  "hAcc"
  v_Acc_m/1 -> Bus Creator/6  "vAcc"
  s_Acc_mDs/1 -> Bus Creator/7  "sAcc"
  Bus Creator/1 -> GPS_Raw/1

== system Plant/Sensor_Model/Sensor_GPS/GPS/Physical_Model ==
  note: Transfer Delay
  States : Inport
  Bus Selector : BusSelector  OutputSignals=Plant_States.lon,Plant_States.lat,Plant_States.alt
  Bus Selector1 : BusSelector  OutputSignals=Plant_States.vel_x_O,Plant_States.vel_y_O,Plant_States.vel_z_O
  Delay : Delay  DelayLength=150/(PLANT_CONST.dt*1e3)
  Delay1 : Delay  DelayLength=100/(PLANT_CONST.dt*1e3)
  Vector Concatenate : Concatenate  NumInputs=3  Mode=Multidimensional array
  Vector Concatenate1 : Concatenate  NumInputs=3  Mode=Multidimensional array
  WGS84_pos_rad : Outport  Unit=rad/s  VectorParamsAs1DForOutWhenUnconnected=off
  vel_O_mPs : Outport  Port=2  Unit=m/s  PortDimensions=[3 1]  VectorParamsAs1DForOutWhenUnconnected=off
  wires:
  Bus Selector/3 -> Vector Concatenate/3  "<alt>"
  Bus Selector/2 -> Vector Concatenate/2  "<lat>"
  Bus Selector/1 -> Vector Concatenate/1  "<lon>"
  Vector Concatenate/1 -> Delay/1
  Bus Selector1/2 -> Vector Concatenate1/2  "<vel_y_O>"
  Bus Selector1/3 -> Vector Concatenate1/3  "<vel_z_O>"
  States/1 -> Bus Selector1/1, Bus Selector/1
  Vector Concatenate1/1 -> Delay1/1
  Bus Selector1/1 -> Vector Concatenate1/1  "<vel_x_O>"
  Delay/1 -> WGS84_pos_rad/1
  Delay1/1 -> vel_O_mPs/1

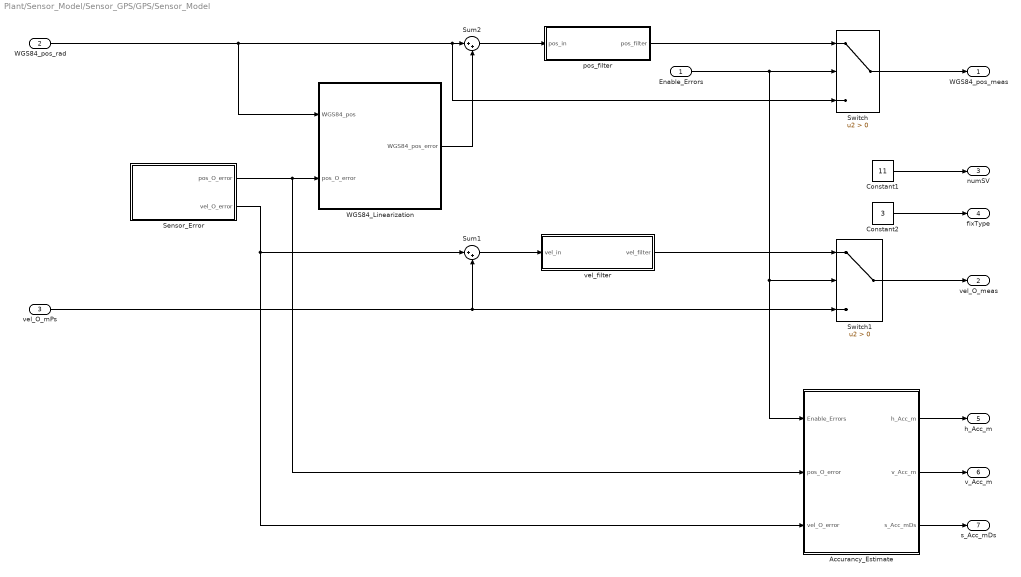
== system Plant/Sensor_Model/Sensor_GPS/GPS/Sensor_Model ==
  Enable_Errors : Inport
  WGS84_pos_rad : Inport  Port=2
  vel_O_mPs : Inport  Port=3
  Accurancy_Estimate : Subsystem
  Constant1 : Constant  Value=11  OutDataTypeStr=Inherit: Inherit via back propagation
  Constant2 : Constant  Value=3  OutDataTypeStr=Inherit: Inherit via back propagation
  Sensor_Error : Subsystem
  Sum1 : Sum  Inputs=|++
  Sum2 : Sum  Inputs=|++
  Switch : Switch  Criteria=u2 > Threshold  SaturateOnIntegerOverflow=off  InputSameDT=off
  Switch1 : Switch  Criteria=u2 > Threshold  SaturateOnIntegerOverflow=off  InputSameDT=off
  WGS84_Linearization : Subsystem
  pos_filter : Subsystem
  vel_filter : Subsystem
  WGS84_pos_meas : Outport  VectorParamsAs1DForOutWhenUnconnected=off
  vel_O_meas : Outport  Port=2  VectorParamsAs1DForOutWhenUnconnected=off
  numSV : Outport  Port=3  VectorParamsAs1DForOutWhenUnconnected=off
  fixType : Outport  Port=4  VectorParamsAs1DForOutWhenUnconnected=off
  h_Acc_m : Outport  Port=5  VectorParamsAs1DForOutWhenUnconnected=off
  v_Acc_m : Outport  Port=6  VectorParamsAs1DForOutWhenUnconnected=off
  s_Acc_mDs : Outport  Port=7  VectorParamsAs1DForOutWhenUnconnected=off
  wires:
  Constant2/1 -> fixType/1
  Constant1/1 -> numSV/1
  Switch/1 -> WGS84_pos_meas/1
  Switch1/1 -> vel_O_meas/1
  Sum2/1 -> pos_filter/1(pos_in)
  Sensor_Error/1(pos_O_error) -> Accurancy_Estimate/2(pos_O_error), WGS84_Linearization/2(pos_O_error)
  Sum1/1 -> vel_filter/1(vel_in)
  Sensor_Error/2(vel_O_error) -> Accurancy_Estimate/3(vel_O_error), Sum1/1
  WGS84_Linearization/1(WGS84_pos_error) -> Sum2/2
  Accurancy_Estimate/1(h_Acc_m) -> h_Acc_m/1
  Accurancy_Estimate/3(s_Acc_mDs) -> s_Acc_mDs/1
  Accurancy_Estimate/2(v_Acc_m) -> v_Acc_m/1
  pos_filter/1(pos_filter) -> Switch/1
  WGS84_pos_rad/1 -> Switch/3, Sum2/1, WGS84_Linearization/1(WGS84_pos)
  vel_O_mPs/1 -> Switch1/3, Sum1/2
  vel_filter/1(vel_filter) -> Switch1/1
  Enable_Errors/1 -> Switch/2, Accurancy_Estimate/1(Enable_Errors), Switch1/2

== system Plant/Sensor_Model/Sensor_IMU/Accelerometer/Bus_Constructor ==
  Output : Inport
  Bus Creator : BusCreator  Inputs=3
  Demux : Demux  Outputs=3
  Acc_Raw : Outport  VectorParamsAs1DForOutWhenUnconnected=off
  wires:
  Demux/2 -> Bus Creator/2  "Acc_y_mPs2"
  Demux/3 -> Bus Creator/3  "Acc_z_mPs2"
  Demux/1 -> Bus Creator/1  "Acc_x_mPs2"
  Bus Creator/1 -> Acc_Raw/1
  Output/1 -> Demux/1

== system Plant/Sensor_Model/Sensor_IMU/Accelerometer/Physical_Model ==
  States : Inport
  specific_force : Subsystem
  sfor_B_mPs2 : Outport  Unit=m/s^2  VectorParamsAs1DForOutWhenUnconnected=off
  wires:
  States/1 -> specific_force/1(States)
  specific_force/1(sfor_B_mPs2) -> sfor_B_mPs2/1

== system Plant/Sensor_Model/Sensor_IMU/Accelerometer/Sensor_Model ==
  Enable_Errors : Inport
  u : Inport  Port=2
  First Order LPF : FMT_Model_Lib/Filter/First Order LPF  fc=Sensor_Model.Acc.Cutoff_frequency_Hz
      settings: SourceProductName=FMT Toolbox
  Saturation : Saturate  UpperLimit=Sensor_Model.Acc.Upper_limit  LowerLimit=Sensor_Model.Acc.Lower_limit
  Sensor_Error : Subsystem
  Sensor_Noise : Subsystem
  Sum : Sum  Inputs=|++
  Switch : Switch  Criteria=u2 > Threshold  SaturateOnIntegerOverflow=off  InputSameDT=off
  y : Outport  VectorParamsAs1DForOutWhenUnconnected=off
  wires:
  Switch/1 -> y/1
  Saturation/1 -> Sum/1
  First Order LPF/1 -> Saturation/1
  Sensor_Error/1(y) -> First Order LPF/1
  Sensor_Noise/1(noise) -> Sum/2
  Enable_Errors/1 -> Switch/2
  u/1 -> Switch/3, Sensor_Error/1(u)
  Sum/1 -> Switch/1

== system Plant/Sensor_Model/Sensor_IMU/Gyroscope/Bus_Constructor ==
  Output : Inport
  Bus Creator : BusCreator  Inputs=3
  Demux : Demux  Outputs=3
  Gyro_Raw : Outport  VectorParamsAs1DForOutWhenUnconnected=off
  wires:
  Demux/1 -> Bus Creator/1  "Gyro_x_radPs"
  Demux/2 -> Bus Creator/2  "Gyro_y_radPs"
  Demux/3 -> Bus Creator/3  "Gyro_z_radPs"
  Bus Creator/1 -> Gyro_Raw/1
  Output/1 -> Demux/1

== system Plant/Sensor_Model/Sensor_IMU/Gyroscope/Physical_Model ==
  States : Inport
  rotation_speed : Subsystem
  gyr_B_radDs : Outport  Unit=rad/s  VectorParamsAs1DForOutWhenUnconnected=off
  wires:
  States/1 -> rotation_speed/1(States)
  rotation_speed/1(rot_radPs) -> gyr_B_radDs/1

== system Plant/Sensor_Model/Sensor_IMU/Gyroscope/Sensor_Model ==
  Enable_Errors : Inport
  u : Inport  Port=2
  First Order LPF : FMT_Model_Lib/Filter/First Order LPF  fc=Sensor_Model.Gyro.Cutoff_frequency_Hz
      settings: SourceProductName=FMT Toolbox
  Saturation : Saturate  UpperLimit=Sensor_Model.Gyro.Range  LowerLimit=-Sensor_Model.Gyro.Range
  Sensor_Error : Subsystem
  Sensor_Noise : Subsystem
  Sum : Sum  Inputs=|++
  Switch : Switch  Criteria=u2 > Threshold  SaturateOnIntegerOverflow=off  InputSameDT=off
  y : Outport  VectorParamsAs1DForOutWhenUnconnected=off
  wires:
  Switch/1 -> y/1
  Saturation/1 -> Sum/1
  First Order LPF/1 -> Saturation/1
  Sensor_Error/1(y) -> First Order LPF/1
  Sensor_Noise/1(noise) -> Sum/2
  Enable_Errors/1 -> Switch/2
  u/1 -> Switch/3, Sensor_Error/1(u)
  Sum/1 -> Switch/1

== system Plant/Sensor_Model/Sensor_MAG/Magnetometer/Bus_Constructor ==
  Output : Inport
  Bus Creator : BusCreator  Inputs=3
  Demux : Demux  Outputs=3
  Mag_Raw : Outport  VectorParamsAs1DForOutWhenUnconnected=off
  wires:
  Demux/2 -> Bus Creator/2  "Mag_y_gauss"
  Demux/1 -> Bus Creator/1  "Mag_x_gauss"
  Bus Creator/1 -> Mag_Raw/1
  Demux/3 -> Bus Creator/3  "Mag_z_gauss"
  Output/1 -> Demux/1

== system Plant/Sensor_Model/Sensor_MAG/Magnetometer/Physical_Model ==
  States : Inport
  Bus Selector : BusSelector  OutputSignals=Plant_States.lat,Plant_States.lon
  Bus Selector1 : BusSelector  OutputSignals=Extended_States.M_BO
  Product : Product  Multiplication=Matrix(*)  InputSameDT=on  RndMeth=Zero  OutDataTypeStr=Inherit: Same as first input
  WMM_LUT : Subsystem  mask{wmm_magnitude=Sensor_Model.Mag.WMM_Mag, wmm_declination=Sensor_Model.Mag.WMM_Dec, wmm_inclination=Sensor_Model.Mag.WMM_Inc, resolution=10}
      mask prompts: wmm_magnitude "WMM Magnitude Lookup Table"; wmm_declination "WMM Declination Lookup Table"; wmm_inclination "WMM Inclination Lookup Table"; resolution "Resolution (deg)"
  magnetic_field : Subsystem
  mag_B_gauss : Outport  Unit=T  PortDimensions=[3 1]  VectorParamsAs1DForOutWhenUnconnected=off
  wires:
  States/1 -> Bus Selector1/1, Bus Selector/1
  Bus Selector/2 -> WMM_LUT/2(lon_rad)  "<lon>"
  Bus Selector/1 -> WMM_LUT/1(lat_rad)  "<lat>"
  Bus Selector1/1 -> Product/1  "<M_BO>"
  Product/1 -> mag_B_gauss/1
  magnetic_field/1(mag_O_gauss) -> Product/2
  WMM_LUT/1(magnitude_uT) -> magnetic_field/1(magnitude_uT)
  WMM_LUT/2(declination_deg) -> magnetic_field/2(declination_deg)
  WMM_LUT/3(inclination_deg) -> magnetic_field/3(inclination_deg)

== system Plant/Sensor_Model/Sensor_MAG/Magnetometer/Sensor_Model ==
  Enable_Errors : Inport
  u : Inport  Port=2
  Add : Sum  InputSameDT=on  OutDataTypeStr=Inherit: Same as first input
  Saturation : Saturate  UpperLimit=Sensor_Model.Mag.Upper_limit  LowerLimit=Sensor_Model.Mag.Lower_limit
  Sensor_Error : Subsystem
  Sensor_Noise : Subsystem
  Switch : Switch  Criteria=u2 > Threshold  SaturateOnIntegerOverflow=off  InputSameDT=off
  y : Outport  VectorParamsAs1DForOutWhenUnconnected=off
  wires:
  Switch/1 -> y/1
  Saturation/1 -> Add/1
  Sensor_Error/1(y) -> Saturation/1
  Sensor_Noise/1(noise) -> Add/2
  Enable_Errors/1 -> Switch/2
  u/1 -> Switch/3, Sensor_Error/1(u)
  Add/1 -> Switch/1

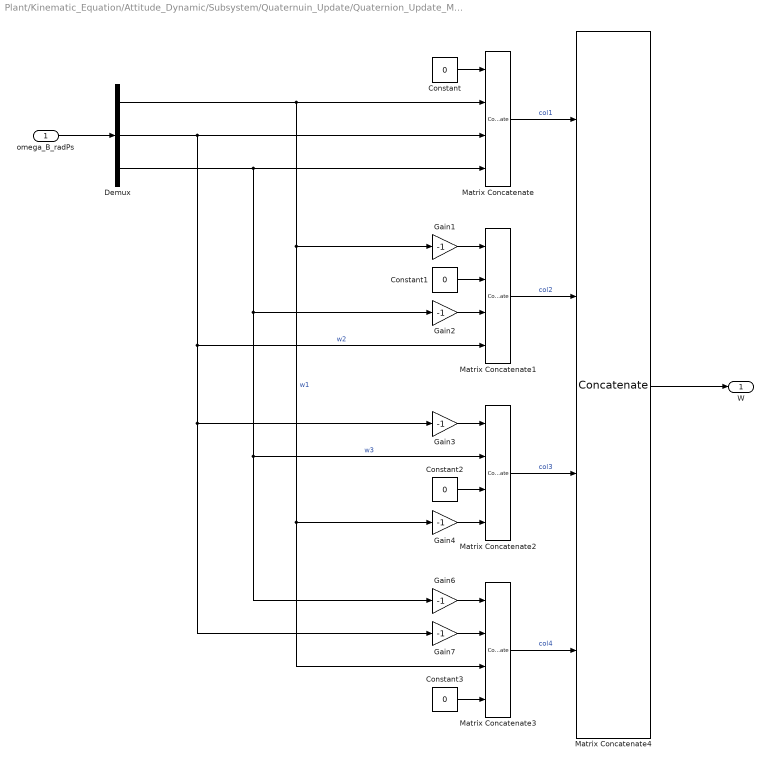
== system Plant/Kinematic_Equation/Attitude_Dynamic/Subsystem/Quaternuin_Update/Quaternion_Update_Maxtrix ==
  omega_B_radPs : Inport
  Constant{,1..3} (4 alike) : Constant  Value=0  OutDataTypeStr=single
  Demux : Demux  Outputs=3
  Gain{1..4,6..7} (6 alike) : Gain  Gain=-1  OutDataTypeStr=Inherit: Same as input
  Matrix Concatenate{,1..3} (4 alike) : Concatenate  NumInputs=4
  Matrix Concatenate4 : Concatenate  NumInputs=4  Mode=Multidimensional array  ConcatenateDimension=2
  W : Outport  VectorParamsAs1DForOutWhenUnconnected=off
  wires:
  Gain1/1 -> Matrix Concatenate1/1
  Gain7/1 -> Matrix Concatenate3/2
  Matrix Concatenate2/1 -> Matrix Concatenate4/3  "col3"
  Constant2/1 -> Matrix Concatenate2/3
  Matrix Concatenate4/1 -> W/1
  Demux/1 -> Matrix Concatenate/2, Gain1/1, Gain4/1, Matrix Concatenate3/3  "w1"
  Matrix Concatenate/1 -> Matrix Concatenate4/1  "col1"
  Matrix Concatenate1/1 -> Matrix Concatenate4/2  "col2"
  Constant3/1 -> Matrix Concatenate3/4
  Gain6/1 -> Matrix Concatenate3/1
  Constant1/1 -> Matrix Concatenate1/2
  Matrix Concatenate3/1 -> Matrix Concatenate4/4  "col4"
  Demux/2 -> Matrix Concatenate1/4, Gain3/1, Gain7/1, Matrix Concatenate/3  "w2"
  Constant/1 -> Matrix Concatenate/1
  Gain3/1 -> Matrix Concatenate2/1
  Demux/3 -> Gain2/1, Matrix Concatenate2/2, Gain6/1, Matrix Concatenate/4  "w3"
  Gain2/1 -> Matrix Concatenate1/3
  omega_B_radPs/1 -> Demux/1
  Gain4/1 -> Matrix Concatenate2/4

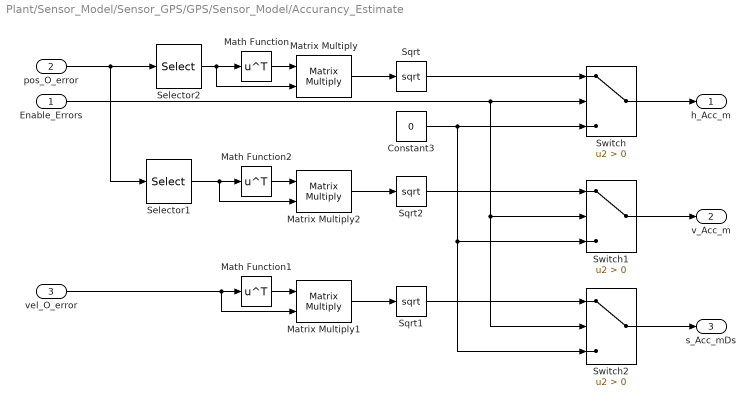
== system Plant/Sensor_Model/Sensor_GPS/GPS/Sensor_Model/Accurancy_Estimate ==
  Enable_Errors : Inport
  pos_O_error : Inport  Port=2
  vel_O_error : Inport  Port=3
  Constant3 : Constant  Value=0
  Math Function : Math  Operator=transpose  SignedPower=on
  Math Function1 : Math  Operator=transpose  SignedPower=on
  Math Function2 : Math  Operator=transpose  SignedPower=on
  Matrix Multiply : Product  Multiplication=Matrix(*)
  Matrix Multiply1 : Product  Multiplication=Matrix(*)
  Matrix Multiply2 : Product  Multiplication=Matrix(*)
  Selector1 : Selector  InputPortWidth=3  IndexOptions=Index vector (dialog)  Indices=3  OutputSizes=1
  Selector2 : Selector  InputPortWidth=3  IndexOptions=Index vector (dialog)  Indices=[1 2]  OutputSizes=1
  Sqrt : Sqrt  OutputSignalType=real
  Sqrt1 : Sqrt  OutputSignalType=real
  Sqrt2 : Sqrt  OutputSignalType=real
  Switch : Switch  Criteria=u2 > Threshold  SaturateOnIntegerOverflow=off  InputSameDT=off
  Switch1 : Switch  Criteria=u2 > Threshold  SaturateOnIntegerOverflow=off  InputSameDT=off
  Switch2 : Switch  Criteria=u2 > Threshold  SaturateOnIntegerOverflow=off  InputSameDT=off
  h_Acc_m : Outport  VectorParamsAs1DForOutWhenUnconnected=off
  v_Acc_m : Outport  Port=2  VectorParamsAs1DForOutWhenUnconnected=off
  s_Acc_mDs : Outport  Port=3  VectorParamsAs1DForOutWhenUnconnected=off
  wires:
  Switch/1 -> h_Acc_m/1
  pos_O_error/1 -> Selector1/1, Selector2/1
  Switch1/1 -> v_Acc_m/1
  Selector1/1 -> Math Function2/1, Matrix Multiply2/2
  Switch2/1 -> s_Acc_mDs/1
  Math Function1/1 -> Matrix Multiply1/1
  Math Function2/1 -> Matrix Multiply2/1
  Math Function/1 -> Matrix Multiply/1
  Selector2/1 -> Matrix Multiply/2, Math Function/1
  Matrix Multiply1/1 -> Sqrt1/1
  Matrix Multiply/1 -> Sqrt/1
  Matrix Multiply2/1 -> Sqrt2/1
  vel_O_error/1 -> Matrix Multiply1/2, Math Function1/1
  Sqrt/1 -> Switch/1
  Sqrt2/1 -> Switch1/1
  Enable_Errors/1 -> Switch2/2, Switch1/2, Switch/2
  Sqrt1/1 -> Switch2/1
  Constant3/1 -> Switch2/3, Switch1/3, Switch/3

== system Plant/Sensor_Model/Sensor_GPS/GPS/Sensor_Model/Sensor_Error ==
  Random Source : dspsrcs4/Random Source  SrcType=Gaussian  NormMethod=Ziggurat  CltLength=12  MinVal=0  MaxVal=1  MeanVal=0  VarVal=[0.02;0.02;0.04].^2  RepMode=Repeatable  rawSeed=1  IsInherit=off  SampMode=Discrete  SampTime=-1  SampFrame=1  DataType=Single  OutComplex=Real  OutputFrames=off
  Random Source1 : dspsrcs4/Random Source  SrcType=Gaussian  NormMethod=Ziggurat  CltLength=12  MinVal=0  MaxVal=1  MeanVal=0  VarVal=[0.01;0.01;0.01].^2  RepMode=Repeatable  rawSeed=1  IsInherit=off  SampMode=Discrete  SampTime=-1  SampFrame=1  DataType=Single  OutComplex=Real  OutputFrames=off
  pos_O_error : Outport  VectorParamsAs1DForOutWhenUnconnected=off
  vel_O_error : Outport  Port=2  VectorParamsAs1DForOutWhenUnconnected=off
  wires:
  Random Source/1 -> pos_O_error/1
  Random Source1/1 -> vel_O_error/1

== system Plant/Sensor_Model/Sensor_GPS/GPS/Sensor_Model/WGS84_Linearization ==
  WGS84_pos : Inport
  pos_O_error : Inport  Port=2
  Demux2 : Demux  Outputs=3
  Divide2 : Product  Inputs=/*
  LAT2FLAT Curve : FMT_Model_Lib/Transformation/LAT2FLAT Curve
      settings: SourceProductName=FMT Toolbox
  Terminator1 : Terminator
  Terminator2 : Terminator
  Vector Concatenate2 : Concatenate  NumInputs=3  Mode=Multidimensional array
  constant1 : Constant  Value=-1
  WGS84_pos_error : Outport  VectorParamsAs1DForOutWhenUnconnected=off
  wires:
  WGS84_pos/1 -> Demux2/1
  Demux2/1 -> LAT2FLAT Curve/1
  LAT2FLAT Curve/2 -> Vector Concatenate2/2
  pos_O_error/1 -> Divide2/2
  Vector Concatenate2/1 -> Divide2/1
  LAT2FLAT Curve/1 -> Vector Concatenate2/1
  Demux2/2 -> Terminator2/1
  Demux2/3 -> Terminator1/1
  constant1/1 -> Vector Concatenate2/3
  Divide2/1 -> WGS84_pos_error/1

== system Plant/Sensor_Model/Sensor_GPS/GPS/Sensor_Model/pos_filter ==
  pos_in : Inport
  Discrete FIR Filter : DiscreteFir
  pos_filter : Outport  VectorParamsAs1DForOutWhenUnconnected=off
  wires:
  Discrete FIR Filter/1 -> pos_filter/1
  pos_in/1 -> Discrete FIR Filter/1

== system Plant/Sensor_Model/Sensor_GPS/GPS/Sensor_Model/vel_filter ==
  vel_in : Inport
  Discrete FIR Filter : DiscreteFir
  vel_filter : Outport  VectorParamsAs1DForOutWhenUnconnected=off
  wires:
  Discrete FIR Filter/1 -> vel_filter/1
  vel_in/1 -> Discrete FIR Filter/1

== system Plant/Sensor_Model/Sensor_IMU/Accelerometer/Physical_Model/specific_force ==
  States : Inport
  Bus Selector : BusSelector  OutputSignals=Plant_States.acc_x_O,Plant_States.acc_y_O,Plant_States.acc_z_O
  Bus Selector1 : BusSelector  OutputSignals=Extended_States.M_BO
  Gravity : Constant  Value=[0;0;Sensor_Model.g]  OutDataTypeStr=single
  Product1 : Product  Multiplication=Matrix(*)  InputSameDT=on  RndMeth=Zero  OutDataTypeStr=Inherit: Same as first input
  Sum : Sum  Inputs=|+-  InputSameDT=on  OutDataTypeStr=Inherit: Same as first input
  Vector Concatenate1 : Concatenate  NumInputs=3  Mode=Multidimensional array
  sfor_B_mPs2 : Outport  Unit=m/s^2  VectorParamsAs1DForOutWhenUnconnected=off
  wires:
  States/1 -> Bus Selector1/1, Bus Selector/1
  Bus Selector/1 -> Vector Concatenate1/1  "<acc_x_O>"
  Bus Selector/2 -> Vector Concatenate1/2  "<acc_y_O>"
  Bus Selector/3 -> Vector Concatenate1/3  "<acc_z_O>"
  Product1/1 -> sfor_B_mPs2/1
  Bus Selector1/1 -> Product1/1  "<M_BO>"
  Vector Concatenate1/1 -> Sum/1
  Sum/1 -> Product1/2
  Gravity/1 -> Sum/2

== system Plant/Sensor_Model/Sensor_IMU/Accelerometer/Sensor_Model/Sensor_Error ==
  u : Inport
  Add : Sum  InputSameDT=on  OutDataTypeStr=Inherit: Same as first input
  Constant : Constant  Value=eye(3)  OutDataTypeStr=single
  Constant1 : Constant  Value=Sensor_Model.Acc.Scalefactor_Error  VectorParams1D=off  OutDataTypeStr=single
  Constant3 : Constant  Value=Sensor_Model.Acc.Bias  VectorParams1D=off  OutDataTypeStr=single
  Product : Product  Multiplication=Matrix(*)  InputSameDT=on  RndMeth=Zero  OutDataTypeStr=Inherit: Same as first input
  Sum : Sum  Inputs=|++  InputSameDT=on  OutDataTypeStr=Inherit: Same as first input
  y : Outport  VectorParamsAs1DForOutWhenUnconnected=off
  wires:
  Sum/1 -> y/1
  Add/1 -> Product/1
  u/1 -> Product/2
  Constant1/1 -> Add/2
  Constant/1 -> Add/1
  Product/1 -> Sum/1
  Constant3/1 -> Sum/2

== system Plant/Sensor_Model/Sensor_IMU/Accelerometer/Sensor_Model/Sensor_Noise ==
  Random Source : dspsrcs4/Random Source  SrcType=Gaussian  NormMethod=Ziggurat  CltLength=12  MinVal=0  MaxVal=1  MeanVal=0  VarVal=Sensor_Model.Acc.Variance  RepMode=Repeatable  rawSeed=1  IsInherit=off  SampMode=Discrete  SampTime=-1  SampFrame=1  DataType=Single  OutComplex=Real  OutputFrames=off
  noise : Outport  VectorParamsAs1DForOutWhenUnconnected=off
  wires:
  Random Source/1 -> noise/1

== system Plant/Sensor_Model/Sensor_IMU/Gyroscope/Physical_Model/rotation_speed ==
  States : Inport
  Bus Selector2 : BusSelector  OutputSignals=Plant_States.rot_x_B,Plant_States.rot_y_B,Plant_States.rot_z_B
  Vector Concatenate : Concatenate  NumInputs=3  Mode=Multidimensional array
  rot_radPs : Outport  VectorParamsAs1DForOutWhenUnconnected=off
  wires:
  Vector Concatenate/1 -> rot_radPs/1
  Bus Selector2/3 -> Vector Concatenate/3  "<rot_z_B>"
  Bus Selector2/1 -> Vector Concatenate/1  "<rot_x_B>"
  Bus Selector2/2 -> Vector Concatenate/2  "<rot_y_B>"
  States/1 -> Bus Selector2/1

== system Plant/Sensor_Model/Sensor_IMU/Gyroscope/Sensor_Model/Sensor_Error ==
  u : Inport
  Add : Sum  InputSameDT=on  OutDataTypeStr=Inherit: Same as first input
  Constant1 : Constant  Value=Sensor_Model.Gyro.Scalefactor_Error  VectorParams1D=off  OutDataTypeStr=single
  Constant2 : Constant  Value=eye(3)  OutDataTypeStr=single
  Constant3 : Constant  Value=Sensor_Model.Gyro.Bias  VectorParams1D=off  OutDataTypeStr=single
  Product : Product  Multiplication=Matrix(*)  InputSameDT=on  RndMeth=Zero  OutDataTypeStr=Inherit: Same as first input
  Sum : Sum  Inputs=|++  InputSameDT=on  OutDataTypeStr=Inherit: Same as first input
  y : Outport  VectorParamsAs1DForOutWhenUnconnected=off
  wires:
  Sum/1 -> y/1
  Product/1 -> Sum/1
  u/1 -> Product/2
  Add/1 -> Product/1
  Constant1/1 -> Add/2
  Constant2/1 -> Add/1
  Constant3/1 -> Sum/2

== system Plant/Sensor_Model/Sensor_IMU/Gyroscope/Sensor_Model/Sensor_Noise ==
  Random Source : dspsrcs4/Random Source  SrcType=Gaussian  NormMethod=Ziggurat  CltLength=12  MinVal=0  MaxVal=1  MeanVal=0  VarVal=Sensor_Model.Gyro.Variance  RepMode=Repeatable  rawSeed=1  IsInherit=off  SampMode=Discrete  SampTime=-1  SampFrame=1  DataType=Single  OutComplex=Real  OutputFrames=off
  noise : Outport  VectorParamsAs1DForOutWhenUnconnected=off
  wires:
  Random Source/1 -> noise/1
